simulink model "control_motor"  (R2023b)
settings: Solver=FixedStepAuto  StartTime=0.0  StopTime=5  RelTol=1e-3  EnableMultiTasking=on
undefined symbols (not defined in the file or in its folder): C, Kid, Ld, sysd, T
libraries: mbedblockslib x6, simulink x2
settings Model: ExtModeTrigDuration=10  Creator=erwinplanck  LastModifiedBy=miqui
settings OptimizationCC: EnhancedBackFolding=on  PassReuseOutputArgsAs=Individual arguments  ZeroExternalMemoryAtStartup=off  ZeroInternalMemoryAtStartup=off  MaxStackSize=64  OptimizeBlockOrder=speed  DifferentSizesBufferReuse=on  OptimizationCustomize=off  EfficientTunableParamExpr=on
settings DebuggingCC: ParameterTunabilityLossMsg=error
settings HardwareCC: ProdBitPerPointer=32  ProdBitPerSizeT=32  ProdBitPerPtrDiffT=32  ProdLargestAtomicInteger=Long  ProdLargestAtomicFloat=Double  ProdWordSize=32  ProdLongLongMode=on  ProdHWDeviceType=ARM Compatible->ARM Cortex  UseEmbeddedCoderFeatures=off
settings SFSimCC: MATLABDynamicMemAlloc=off
settings RTWCC: Description=Embedded Coder  SystemTargetFile=ert.tlc  HardwareBoard=STM32 Nucleo F411RE  TemplateMakefile=ert_default_tmf  Toolchain=GNU Tools for ARM Embedded Processors
settings CodeAppCC: ForceParamTrailComments=on  IgnoreCustomStorageClasses=off  OperatorAnnotations=on  SimulinkDataObjDesc=on  SFDataObjDesc=on  InsertBlockDesc=on
settings ERTTargetCC: SupportNonInlinedSFcns=on  ExtModeTransport=3  ExtModeStaticAlloc=on  ExtModeStaticAllocSize=2000  ExtModeMexFile=ext_xcp  ExtModeIntrfLevel=Level2 - Open

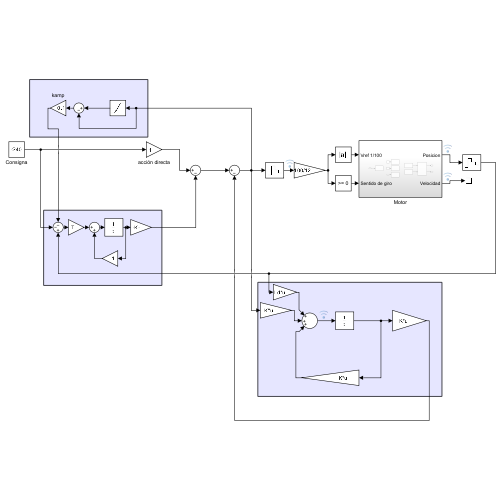
[thumbnail: Simulink's stored preview of the top-level diagram]
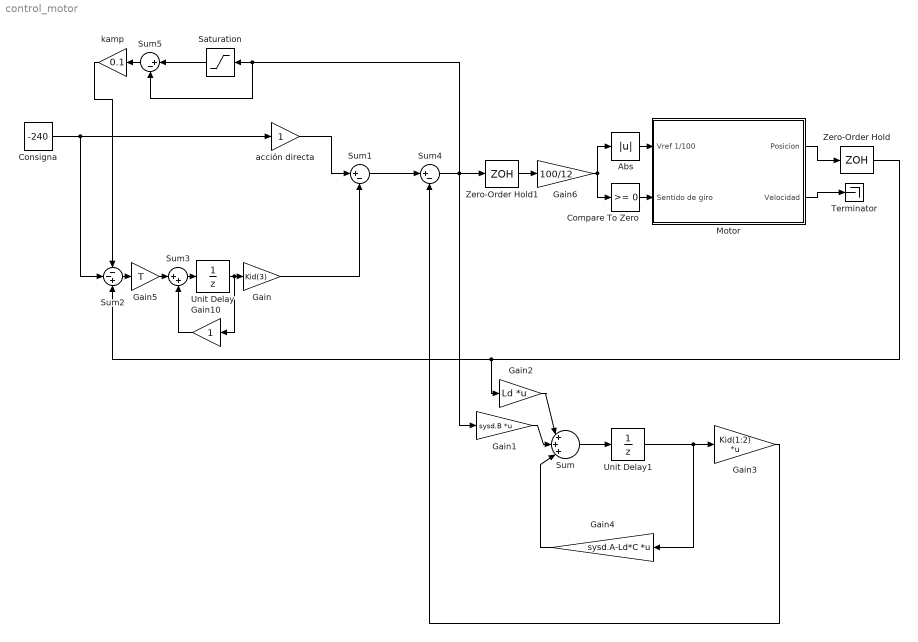
== system control_motor ==
  Abs : Abs  SaturateOnIntegerOverflow=off
  Compare To Zero : simulink/Logic and Bit Operations/Compare To Zero  relop=>=  OutDataTypeStr=boolean
  Consigna : Constant  Value=-240
  Gain : Gain  Gain=Kid(3)
  Gain1 : Gain  Gain=sysd.B  Multiplication=Matrix(K*u)
  Gain10 : Gain
  Gain2 : Gain  Gain=Ld  Multiplication=Matrix(K*u)
  Gain3 : Gain  Gain=Kid(1:2)  Multiplication=Matrix(K*u)
  Gain4 : Gain  Gain=sysd.A-Ld*C  Multiplication=Matrix(K*u)
  Gain5 : Gain  Gain=T
  Gain6 : Gain  Gain=100/12
  Motor : Subsystem
  Saturation : Saturate  UpperLimit=12  LowerLimit=-12
  Sum : Sum  Inputs=|+++|
  Sum1 : Sum  Inputs=|+-
  Sum2 : Sum  Inputs=--+
  Sum3 : Sum  Inputs=|++
  Sum4 : Sum  Inputs=|+-
  Sum5 : Sum  Inputs=|+-
  Terminator : Terminator
  Unit Delay : UnitDelay  SampleTime=T  HasFrameUpgradeWarning=on
  Unit Delay1 : UnitDelay  SampleTime=T  HasFrameUpgradeWarning=on
  Zero-Order Hold : ZeroOrderHold  SampleTime=T
  Zero-Order Hold1 : ZeroOrderHold  SampleTime=T
  acción directa : Gain
  kamp : Gain  Gain=0.1
  wires:
  Zero-Order Hold1/1 -> Gain6/1
  Gain5/1 -> Sum3/1
  Sum4/1 -> Gain1/1, Sum5/2, Saturation/1, Zero-Order Hold1/1
  kamp/1 -> Sum2/1
  Unit Delay/1 -> Gain10/1, Gain/1
  Zero-Order Hold/1 -> Sum2/3, Gain2/1
  Gain2/1 -> Sum/1
  Gain10/1 -> Sum3/2
  Gain1/1 -> Sum/2
  Sum5/1 -> kamp/1
  Unit Delay1/1 -> Gain4/1, Gain3/1
  Saturation/1 -> Sum5/1
  Sum/1 -> Unit Delay1/1
  Motor/2(Velocidad) -> Terminator/1
  Sum2/1 -> Gain5/1
  Sum1/1 -> Sum4/1
  Gain/1 -> Sum1/2
  Consigna/1 -> acción directa/1, Sum2/2
  Gain3/1 -> Sum4/2
  Sum3/1 -> Unit Delay/1
  Gain4/1 -> Sum/3
  Motor/1(Posicion) -> Zero-Order Hold/1
  acción directa/1 -> Sum1/1
  Gain6/1 -> Abs/1, Compare To Zero/1
  Compare To Zero/1 -> Motor/2(Sentido de giro)
  Abs/1 -> Motor/1(Vref 1/100)

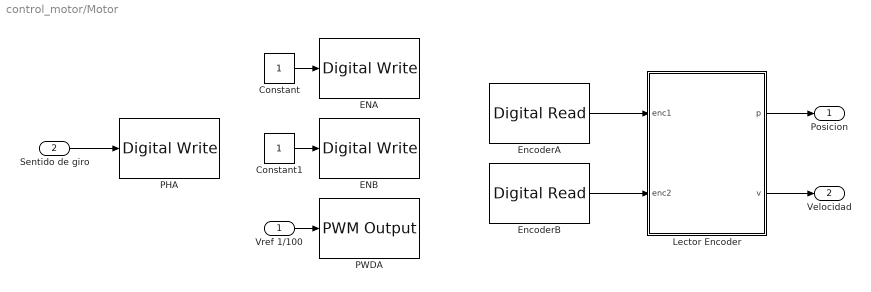
== system control_motor/Motor ==
  Vref 1/100 : Inport
  Sentido de giro : Inport  Port=2
  Constant : Constant
  Constant1 : Constant
  ENA : mbedblockslib/Digital Write  Pin=D2  Direction=output
  ENB : mbedblockslib/Digital Write  Pin=D11  Direction=output
  EncoderA : mbedblockslib/Digital Read  Pin=A1  Direction=input  SampleTime=0.0001
  EncoderB : mbedblockslib/Digital Read  Pin=A0  Direction=input  SampleTime=0.0001
  Lector Encoder : Subsystem
  PHA : mbedblockslib/Digital Write  Pin=D3  Direction=output
  PWDA : mbedblockslib/PWM Output  Pin=D5  EnableInputFrequency=off  InitialFrequency=5000  InitialDutyCycle=0  NotificationType=None
  Posicion : Outport
  Velocidad : Outport  Port=2
  wires:
  Sentido de giro/1 -> PHA/1
  Vref 1/100/1 -> PWDA/1
  Constant/1 -> ENA/1
  Constant1/1 -> ENB/1
  Lector Encoder/1(p) -> Posicion/1
  Lector Encoder/2(v) -> Velocidad/1
  EncoderB/1 -> Lector Encoder/2(enc2)
  EncoderA/1 -> Lector Encoder/1(enc1)

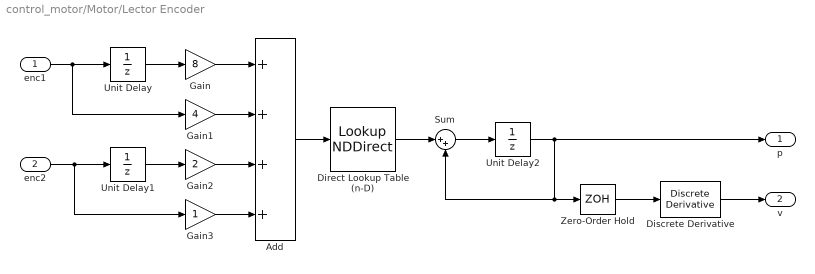
== system control_motor/Motor/Lector Encoder ==
  enc1 : Inport
  enc2 : Inport  Port=2
  Add : Sum  Inputs=++++  OutDataTypeStr=double
  Direct Lookup Table (n-D) : LookupNDDirect  NumberOfTableDimensions=1  Table=[0,-1,1,0,1,0,0,-1,-1,0,0,1,0,1,-1,0]
  Discrete Derivative : simulink/Discrete/Discrete Derivative  gainval=1.0  ICPrevScaledInput=0.0  OutMin=[]  OutMax=[]  OutDataType=fixdt(1, 16)  OutScaling=2^-10  DoSatur=off
  Gain : Gain  Gain=8
  Gain1 : Gain  Gain=4
  Gain2 : Gain  Gain=2
  Gain3 : Gain
  Sum : Sum  Inputs=|++
  Unit Delay : UnitDelay  SampleTime=-1  HasFrameUpgradeWarning=on
  Unit Delay1 : UnitDelay  SampleTime=-1  HasFrameUpgradeWarning=on
  Unit Delay2 : UnitDelay  SampleTime=-1  HasFrameUpgradeWarning=on
  Zero-Order Hold : ZeroOrderHold  SampleTime=0.01
  p : Outport
  v : Outport  Port=2
  wires:
  Zero-Order Hold/1 -> Discrete Derivative/1
  Discrete Derivative/1 -> v/1
  Add/1 -> Direct Lookup Table (n-D)/1
  enc1/1 -> Unit Delay/1, Gain1/1
  Direct Lookup Table (n-D)/1 -> Sum/1
  Gain2/1 -> Add/3
  Gain/1 -> Add/1
  Sum/1 -> Unit Delay2/1
  Unit Delay1/1 -> Gain2/1
  enc2/1 -> Unit Delay1/1, Gain3/1
  Gain1/1 -> Add/2
  Unit Delay/1 -> Gain/1
  Gain3/1 -> Add/4
  Unit Delay2/1 -> Zero-Order Hold/1, Sum/2, p/1
